simulink model "model_closedloop"  (R2019b)
settings: Solver=FixedStepAuto  StartTime=0.0  StopTime=t_end  FixedStep=dt  MaxStep=.1  RelTol=1e-3
values from neighbouring files (symbols this model uses):
  Ts = 30*dt    (= 0.3)    [duffing_init.m]    (also in duffing_linear.m = 10*dt; f_init_hybrid.m = 0.2)
settings Model: Creator=enrique.babio  LastModifiedBy=enrique.babio
settings DataIOCC: ExternalInput=getinputstruct(opTrim)  InitialState=getstatestruct(opTrim)  SaveState=on

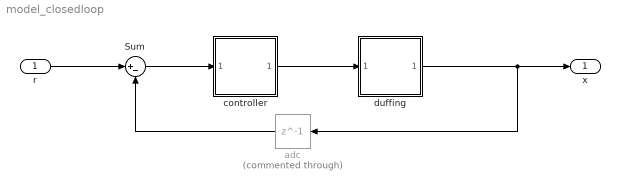
== system model_closedloop ==
  r : Inport
  Sum : Sum  Inputs=|+-
  adc : Delay  Commented=through  DelayLength=1  SampleTime=Ts  StateName=adcDelay
  controller : Subsystem  ReferencedSubsystem=controller
  duffing : Subsystem  ReferencedSubsystem=duffing
  x : Outport
  wires:
  duffing/1 -> adc/1, x/1
  controller/1 -> duffing/1
  r/1 -> Sum/1
  Sum/1 -> controller/1
  adc/1 -> Sum/2
